simulink model "MBD_Design"  (R2018a)
settings: Solver=FixedStepDiscrete  StartTime=0.0  StopTime=inf  RelTol=1e-3  EnableMultiTasking=on
libraries: arduinolib x6
settings Model: SimulationMode=external  ExtModeTrigDuration=2  Creator=vatsald  LastModifiedBy=vatsald
settings OptimizationCC: EnhancedBackFolding=on  PassReuseOutputArgsAs=Individual arguments  MaxStackSize=64  OptimizeBlockOrder=speed  DifferentSizesBufferReuse=on  OptimizationCustomize=off
settings DebuggingCC: ParameterTunabilityLossMsg=error
settings HardwareCC: ProdBitPerInt=16  ProdBitPerPointer=16  ProdBitPerSizeT=16  ProdBitPerPtrDiffT=16  ProdLargestAtomicFloat=None  ProdWordSize=8  ProdHWDeviceType=Atmel->AVR  UseEmbeddedCoderFeatures=off  UseSimulinkCoderFeatures=off
settings SFSimCC: MATLABDynamicMemAlloc=off
settings RTWCC: SystemTargetFile=ert.tlc  HardwareBoard=Arduino Uno  TLCOptions=-aInlineSetEventsForThisBaseRateFcn=TLC_FALSE -aSuppressMultiTaskScheduler=TLC_FALSE -aRateBasedStepFcn=1  TemplateMakefile=ert_default_tmf  GenerateReport=on  Toolchain=Arduino AVR  BuildConfiguration=Faster Runs  IncludeHyperlinkInReport=on  LaunchReport=on  GenerateTraceInfo=on  GenerateTraceReport=on  GenerateTraceReportSl=on  GenerateTraceReportSf=on  GenerateTraceReportEml=on
settings CodeAppCC: ForceParamTrailComments=on  IgnoreCustomStorageClasses=off  OperatorAnnotations=on  SimulinkDataObjDesc=on  SFDataObjDesc=on  MangleLength=10  InsertBlockDesc=on
settings ERTTargetCC: SupportContinuousTime=on  SupportNonInlinedSFcns=on  SupportVariableSizeSignals=on

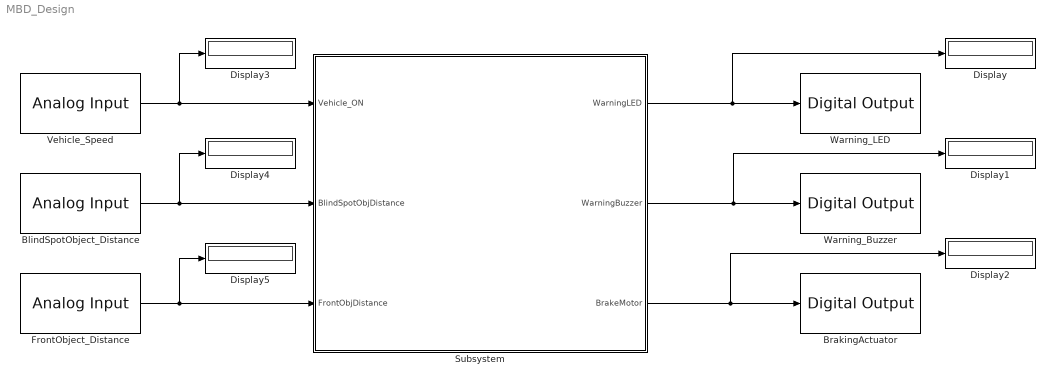
== system MBD_Design ==
  BlindSpotObject_Distance : arduinolib/Analog Input  pinNumber=1  ReadResultsOnly=off  ConversionTriggerSource=Software  ExternalTriggerType=uint32(0)  OutputDataType=uint16  EnableConversionCompleteNotify=off  EnableOuputStatus=off  SampleTime=1  blockPlatform=arduino
  BrakingActuator : arduinolib/Digital Output  pinNumber=3  blockPlatform=arduino
  Display{,1..5} (6 alike) : Display
  FrontObject_Distance : arduinolib/Analog Input  pinNumber=2  ReadResultsOnly=off  ConversionTriggerSource=Software  ExternalTriggerType=uint32(0)  OutputDataType=uint16  EnableConversionCompleteNotify=off  EnableOuputStatus=off  SampleTime=1  blockPlatform=arduino
  Subsystem : Subsystem
  Vehicle_Speed : arduinolib/Analog Input  pinNumber=0  ReadResultsOnly=off  ConversionTriggerSource=Software  ExternalTriggerType=uint32(0)  OutputDataType=uint16  EnableConversionCompleteNotify=off  EnableOuputStatus=off  SampleTime=1  blockPlatform=arduino
  Warning_Buzzer : arduinolib/Digital Output  pinNumber=8  blockPlatform=arduino
  Warning_LED : arduinolib/Digital Output  pinNumber=5  blockPlatform=arduino
  wires:
  Subsystem/3(BrakeMotor) -> Display2/1, BrakingActuator/1
  Subsystem/2(WarningBuzzer) -> Display1/1, Warning_Buzzer/1
  Subsystem/1(WarningLED) -> Display/1, Warning_LED/1
  Vehicle_Speed/1 -> Display3/1, Subsystem/1(Vehicle_ON)
  BlindSpotObject_Distance/1 -> Display4/1, Subsystem/2(BlindSpotObjDistance)
  FrontObject_Distance/1 -> Display5/1, Subsystem/3(FrontObjDistance)

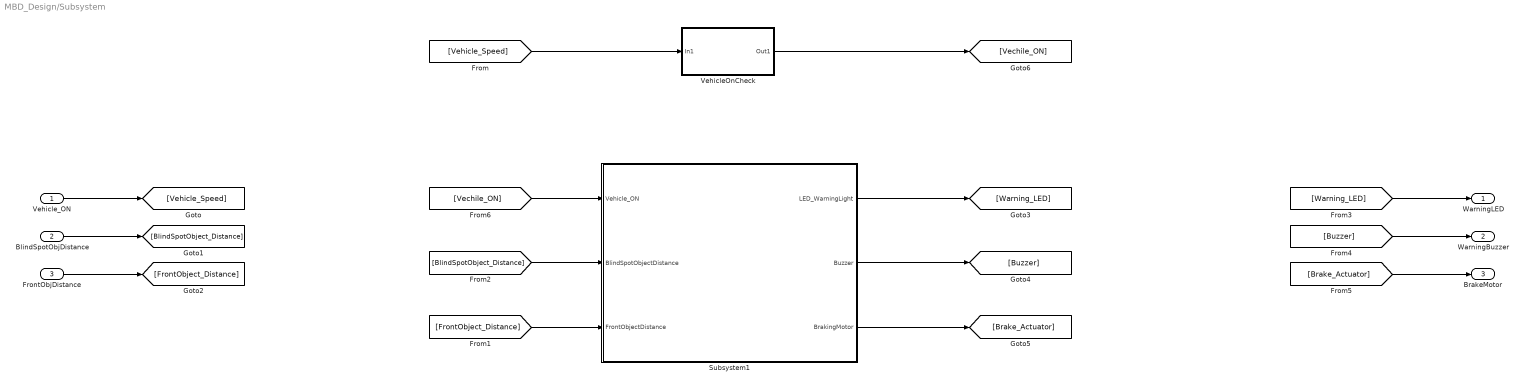
== system MBD_Design/Subsystem ==
  Vehicle_ON : Inport
  BlindSpotObjDistance : Inport  Port=2
  FrontObjDistance : Inport  Port=3
  Subsystem1 : Subsystem
  VehicleOnCheck : Subsystem
  WarningLED : Outport
  WarningBuzzer : Outport  Port=2
  BrakeMotor : Outport  Port=3
  wires:
  [Buzzer] -> WarningBuzzer/1
  [Warning_LED] -> WarningLED/1
  [Brake_Actuator] -> BrakeMotor/1
  Vehicle_ON/1 -> [Vehicle_Speed]
  BlindSpotObjDistance/1 -> [BlindSpotObject_Distance]
  FrontObjDistance/1 -> [FrontObject_Distance]
  [Vehicle_Speed] -> VehicleOnCheck/1(In1)
  VehicleOnCheck/1(Out1) -> [Vechile_ON]
  [Vechile_ON] -> Subsystem1/1(Vehicle_ON)
  [BlindSpotObject_Distance] -> Subsystem1/2(BlindSpotObjectDistance)
  [FrontObject_Distance] -> Subsystem1/3(FrontObjectDistance)
  Subsystem1/3(BrakingMotor) -> [Brake_Actuator]
  Subsystem1/2(Buzzer) -> [Buzzer]
  Subsystem1/1(LED_WarningLight) -> [Warning_LED]

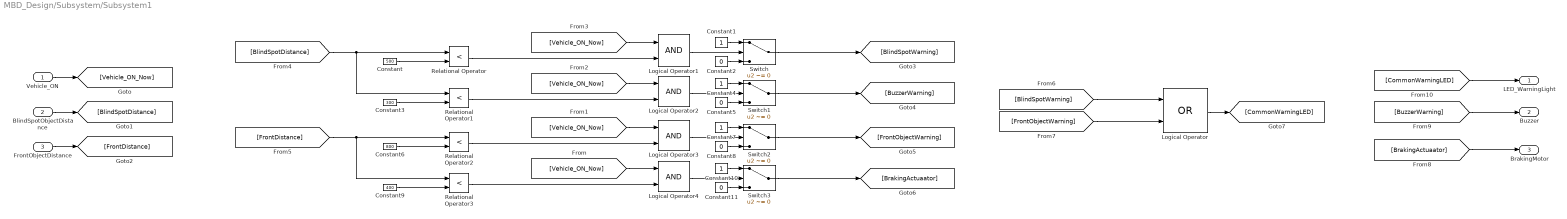
== system MBD_Design/Subsystem/Subsystem1 ==
  Vehicle_ON : Inport
  BlindSpotObjectDistance : Inport  Port=2
  FrontObjectDistance : Inport  Port=3
  Constant : Constant  Value=500
  Constant{1,4,7,10} (4 alike) : Constant
  Constant{2,5,8,11} (4 alike) : Constant  Value=0
  Constant3 : Constant  Value=300
  Constant6 : Constant  Value=800
  Constant9 : Constant  Value=400
  Logical Operator : Logic  Operator=OR  AllPortsSameDT=off  OutDataTypeStr=boolean
  Logical Operator{1..4} (4 alike) : Logic  AllPortsSameDT=off  OutDataTypeStr=boolean
  Relational Operator{,1..3} (4 alike) : RelationalOperator  Operator=<  OutDataTypeStr=boolean  RndMeth=Simplest
  Switch{,1..3} (4 alike) : Switch  Criteria=u2 ~= 0
  LED_WarningLight : Outport
  Buzzer : Outport  Port=2
  BrakingMotor : Outport  Port=3
  wires:
  Constant9/1 -> Relational Operator3/2
  Logical Operator3/1 -> Switch2/2
  [Vehicle_ON_Now] -> Logical Operator4/1
  Relational Operator3/1 -> Logical Operator4/2
  Logical Operator4/1 -> Switch3/2
  Switch3/1 -> [BrakingActuaator]
  Constant3/1 -> Relational Operator1/2
  Switch2/1 -> [FrontObjectWarning]
  Logical Operator1/1 -> Switch/2
  Constant/1 -> Relational Operator/2
  Relational Operator2/1 -> Logical Operator3/2
  Constant2/1 -> Switch/3
  Constant1/1 -> Switch/1
  Logical Operator2/1 -> Switch1/2
  Switch1/1 -> [BuzzerWarning]
  Relational Operator1/1 -> Logical Operator2/2
  Constant4/1 -> Switch1/1
  [FrontDistance] -> Relational Operator3/1, Relational Operator2/1
  Relational Operator/1 -> Logical Operator1/2
  Constant5/1 -> Switch1/3
  [BlindSpotDistance] -> Relational Operator1/1, Relational Operator/1
  Constant6/1 -> Relational Operator2/2
  Constant10/1 -> Switch3/1
  Constant11/1 -> Switch3/3
  Logical Operator/1 -> [CommonWarningLED]
  Constant7/1 -> Switch2/1
  Constant8/1 -> Switch2/3
  Switch/1 -> [BlindSpotWarning]
  Vehicle_ON/1 -> [Vehicle_ON_Now]
  [Vehicle_ON_Now] -> Logical Operator1/1
  [Vehicle_ON_Now] -> Logical Operator2/1
  [Vehicle_ON_Now] -> Logical Operator3/1
  BlindSpotObjectDistance/1 -> [BlindSpotDistance]
  FrontObjectDistance/1 -> [FrontDistance]
  [BlindSpotWarning] -> Logical Operator/1
  [FrontObjectWarning] -> Logical Operator/2
  [CommonWarningLED] -> LED_WarningLight/1
  [BuzzerWarning] -> Buzzer/1
  [BrakingActuaator] -> BrakingMotor/1

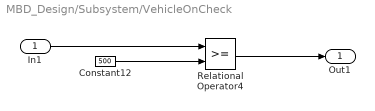
== system MBD_Design/Subsystem/VehicleOnCheck ==
  In1 : Inport
  Constant12 : Constant  Value=500
  Relational Operator4 : RelationalOperator  OutDataTypeStr=boolean  RndMeth=Simplest
  Out1 : Outport
  wires:
  Constant12/1 -> Relational Operator4/2
  Relational Operator4/1 -> Out1/1
  In1/1 -> Relational Operator4/1
